simulink model "sys_model"  (R2021a)
settings: Solver=ode45  StartTime=0.0  StopTime=15  RelTol=1e-3
values from neighbouring files (symbols this model uses):
  b = 50.0    [sys_dict.sldd]
  Ki = 350.0    [sys_dict.sldd]
  Kp = 650.0    [sys_dict.sldd]
  m = 1000.0    [sys_dict.sldd]
  Ts = 0.01    [sys_dict.sldd]
settings Model: DataDictionary=sys_dict.sldd  Creator=Rasika Shejul  LastModifiedBy=Rushikesh
settings SolverCC: AlgebraicLoopSolver=TrustRegion
settings DebuggingCC: SFMachineParentedDataDiag=warning

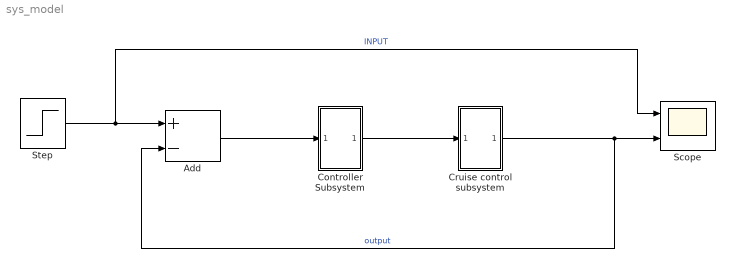
== system sys_model ==
  Add : Sum  Inputs=+-
  Controller Subsystem : Subsystem
  Cruise control subsystem : Subsystem
  Scope : Scope  NumInputPorts=2
  Step : Step  SampleTime=0
  wires:
  Add/1 -> Controller Subsystem/1(In1)
  Controller Subsystem/1(Output) -> Cruise control subsystem/1(Inport)
  Cruise control subsystem/1(Output) -> Add/2, Scope/2  "output"
  Step/1 -> Scope/1, Add/1  "INPUT"

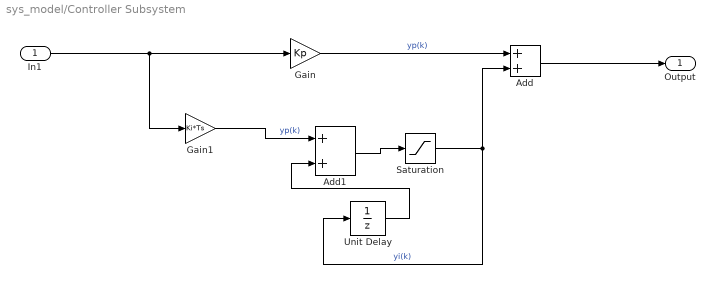
== system sys_model/Controller Subsystem ==
  In1 : Inport
  Add : Sum
  Add1 : Sum
  Gain : Gain  Gain=Kp
  Gain1 : Gain  Gain=Ki*Ts
  Saturation : Saturate  UpperLimit=1  LowerLimit=-1
  Unit Delay : UnitDelay  SampleTime=-1  HasFrameUpgradeWarning=on
  Output : Outport
  wires:
  In1/1 -> Gain1/1, Gain/1
  Gain1/1 -> Add1/1  "yp(k)"
  Unit Delay/1 -> Add1/2
  Add/1 -> Output/1
  Gain/1 -> Add/1  "yp(k)"
  Saturation/1 -> Add/2, Unit Delay/1  "yi(k)"
  Add1/1 -> Saturation/1

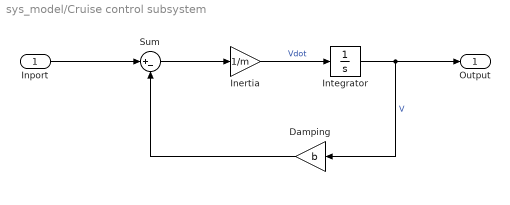
== system sys_model/Cruise control subsystem ==
  Inport : Inport
  Damping : Gain  Gain=b
  Inertia : Gain  Gain=1/m
  Integrator : Integrator
  Sum : Sum  Inputs=|+-
  Output : Outport
  wires:
  Inport/1 -> Sum/1
  Inertia/1 -> Integrator/1  "Vdot"
  Integrator/1 -> Output/1, Damping/1  "V"
  Damping/1 -> Sum/2
  Sum/1 -> Inertia/1
